simulink model "BalanceBotR2016b"  (R2016b)
settings: Solver=FixedStepAuto  StartTime=0.0  StopTime=inf  FixedStep=0.005  RelTol=1e-3
values from neighbouring files (symbols this model uses):
  K = lqr(A,B,Q,R)    [param4BalanceBot.m]
libraries: BrickPi x6
settings Model: SimulationMode=external  Creator=Isshu  LastModifiedBy=Isshu
settings SolverCC: PositivePriorityOrder=on
settings OptimizationCC: EnhancedBackFolding=on  PassReuseOutputArgsAs=Individual arguments  MaxStackSize=64
settings DebuggingCC: ParameterTunabilityLossMsg=error
settings HardwareCC: ProdBitPerPointer=32  ProdBitPerSizeT=32  ProdBitPerPtrDiffT=32  ProdLargestAtomicInteger=Long  ProdLargestAtomicFloat=Double  ProdWordSize=32  ProdHWDeviceType=ARM Compatible->ARM Cortex  UseEmbeddedCoderFeatures=off  UseSimulinkCoderFeatures=off
settings ModelReferenceCC: PropagateVarSize=During execution
settings SFSimCC: SimUseLocalCustomCode=on
settings RTWCC: SystemTargetFile=ert.tlc  HardwareBoard=Raspberry Pi  TLCOptions="-aInlineSetEventsForThisBaseRateFcn=TLC_FALSE -aSuppressMultiTaskScheduler=TLC_FALSE  -aRateBasedStepFcn=0"  TemplateMakefile=ert_default_tmf  Description=Embedded Coder  RTWVerbose=off  RTWUseLocalCustomCode=on  Toolchain=GNU GCC Raspberry Pi  BuildConfiguration=Faster Runs  IncludeHyperlinkInReport=on
settings CodeAppCC: ForceParamTrailComments=on  OperatorAnnotations=on  SimulinkDataObjDesc=on  SFDataObjDesc=on  MangleLength=10  InsertBlockDesc=on
settings ERTTargetCC: MultiwordLength=256  SupportNonInlinedSFcns=on  SupportVariableSizeSignals=on  ExtMode=on  ExtModeMexArgs='169.254.0.2' 0 17725  ERTSrcFileBannerTemplate=codertarget_code_template.cgt  ERTHdrFileBannerTemplate=codertarget_code_template.cgt  ERTDataSrcFileTemplate=codertarget_code_template.cgt  ERTDataHdrFileTemplate=codertarget_code_template.cgt

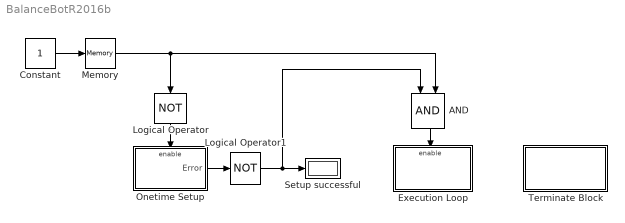
== system BalanceBotR2016b ==
  AND : Logic  AllPortsSameDT=off  OutDataTypeStr=boolean
  Constant : Constant
  Execution Loop : Subsystem
  Logical Operator : Logic  Operator=NOT  AllPortsSameDT=off  OutDataTypeStr=boolean
  Logical Operator1 : Logic  Operator=NOT  AllPortsSameDT=off  OutDataTypeStr=boolean
  Memory : Memory
  Onetime Setup : Subsystem
  Setup successful : Display
  Terminate Block : Subsystem  TreatAsAtomicUnit=on
  wires:
  Constant/1 -> Memory/1
  Logical Operator/1 -> Onetime Setup/Enable
  Onetime Setup/1(Error) -> Logical Operator1/1
  AND/1 -> Execution Loop/Enable
  Logical Operator1/1 -> Setup successful/1, AND/1
  Memory/1 -> AND/2, Logical Operator/1

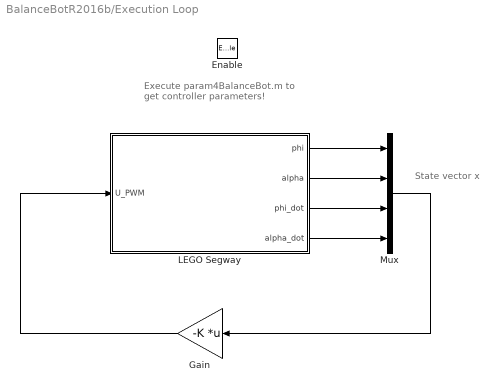
== system BalanceBotR2016b/Execution Loop ==
  note: Execute param4BalanceBot.m to get controller parameters!
  note: State vector x
  Enable : EnablePort
  Gain : Gain  Gain=-K  Multiplication=Matrix(K*u) (u vector)
  LEGO Segway : Subsystem
  Mux : Mux
  wires:
  Mux/1 -> Gain/1
  LEGO Segway/1(phi) -> Mux/1
  Gain/1 -> LEGO Segway/1(U_PWM)
  LEGO Segway/4(alpha_dot) -> Mux/4
  LEGO Segway/2(alpha) -> Mux/2
  LEGO Segway/3(phi_dot) -> Mux/3

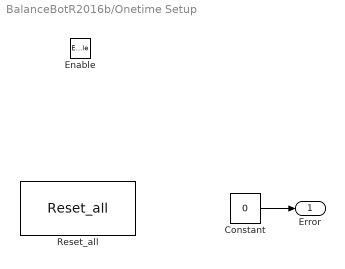
== system BalanceBotR2016b/Onetime Setup ==
  Enable : EnablePort
  Constant : Constant  Value=0
  Reset_all : BrickPi/Reset_all
  Error : Outport  InitialOutput=[1]
  wires:
  Constant/1 -> Error/1

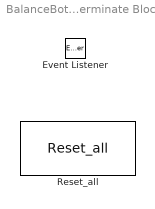
== system BalanceBotR2016b/Terminate Block ==
  Event Listener : EventListener  DisableCoverage=on  EventType=Terminate  EventName=reset
  Reset_all : BrickPi/Reset_all

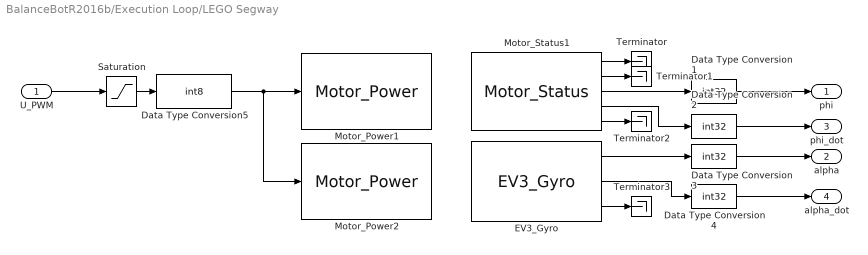
== system BalanceBotR2016b/Execution Loop/LEGO Segway ==
  U_PWM : Inport
  Data Type Conversion{1..4} (4 alike) : DataTypeConversion  OutDataTypeStr=int32
  Data Type Conversion5 : DataTypeConversion  OutDataTypeStr=int8
  EV3_Gyro : BrickPi/EV3_Gyro  SensorPort=4  SensorType=SENSOR_TYPE_EV3_GYRO_ABS_DPS
  Motor_Power1 : BrickPi/Motor_Power  MotorPort=A  choice=Power  Kp=0  Kd=0  Kp_DPS=0  Kd_DPS=0
  Motor_Power2 : BrickPi/Motor_Power  MotorPort=D  choice=Power  Kp=0  Kd=0  Kp_DPS=0  Kd_DPS=0
  Motor_Status1 : BrickPi/Motor_Status  MotorPort=A  ResetMode=Never reset
  Saturation : Saturate  UpperLimit=100  LowerLimit=-100
  Terminator{,1..3} (4 alike) : Terminator
  phi : Outport
  alpha : Outport  Port=2
  phi_dot : Outport  Port=3
  alpha_dot : Outport  Port=4
  wires:
  EV3_Gyro/2 -> Data Type Conversion4/1
  Motor_Status1/4 -> Data Type Conversion2/1
  Motor_Status1/3 -> Data Type Conversion1/1
  EV3_Gyro/1 -> Data Type Conversion3/1
  Data Type Conversion5/1 -> Motor_Power2/1, Motor_Power1/1
  Saturation/1 -> Data Type Conversion5/1
  Motor_Status1/1 -> Terminator/1
  Motor_Status1/2 -> Terminator1/1
  Motor_Status1/5 -> Terminator2/1
  EV3_Gyro/3 -> Terminator3/1
  U_PWM/1 -> Saturation/1
  Data Type Conversion2/1 -> phi_dot/1
  Data Type Conversion1/1 -> phi/1
  Data Type Conversion3/1 -> alpha/1
  Data Type Conversion4/1 -> alpha_dot/1
